simulink model "Open_Ciruit_Tests_of_Single_Phase_Transformer"  (R2025a)
settings: Solver=ode23tb  StartTime=0.0  StopTime=5  MaxStep=1e-4  RelTol=1e-3
libraries: spsRMSLib x2, spsCurrentMeasurementLib x1, spsLinearTransformerLib x1, spsPowerLib x1, spsVoltageMeasurementLib x1, spsACVoltageSourceLib x1, spspowerguiLib x1
settings Model: Creator=Jawad  LastModifiedBy=Jawad

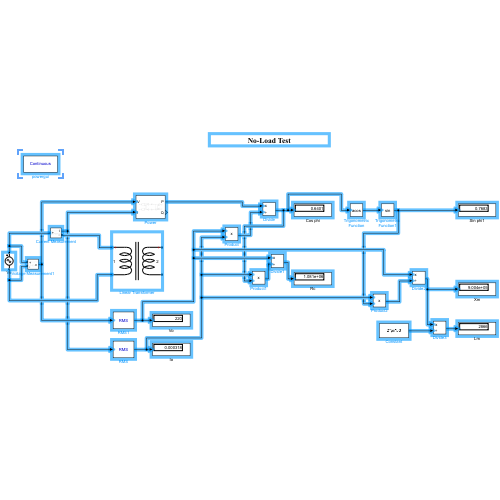
[thumbnail: Simulink's stored preview of the top-level diagram]
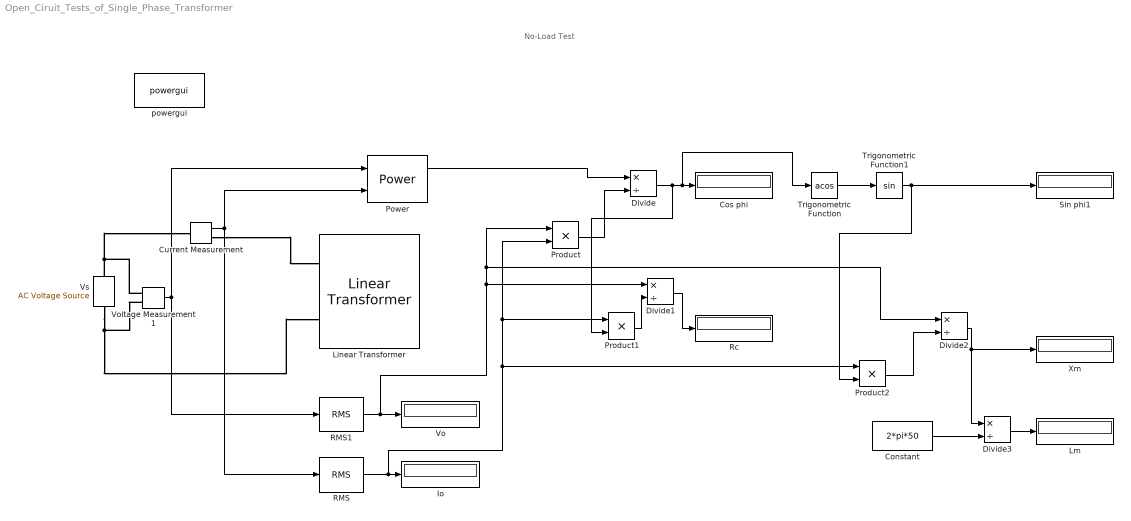
== system Open_Ciruit_Tests_of_Single_Phase_Transformer ==
  note: No-Load Test
  Constant : Constant  Value=2*pi*50
  Cos phi : Display
  Current Measurement : spsCurrentMeasurementLib/Current Measurement  PhasorSimulation=off  OutputType=Complex  PSBequivalent=0
  Divide{,1..3} (4 alike) : Product  Inputs=*/
  Io : Display
  Linear Transformer : spsLinearTransformerLib/Linear Transformer  UNITS=SI  NominalPower=[ 2000 50 ]  winding1=[220 4.3218 0.45856]  winding2=[110 0.7938 0.084225]  ThreeWindings=off  winding3=[3.15e+05 0.7938 0.084225]  RmLm=[1.0804e+06 2866]  Measurements=None  DataType=on
  Lm : Display
  Power : spsPowerLib/Power  Freq=50  Vinit=[1, 0]  Iinit=[1, 0]  Ts=0
  Product : Product
  Product1 : Product
  Product2 : Product
  RMS : spsRMSLib/RMS  TrueRMS=off  Freq=50  RMSInit=0  Ts=0
  RMS1 : spsRMSLib/RMS  TrueRMS=off  Freq=50  RMSInit=0  Ts=0
  Rc : Display
  Sin phi1 : Display
  Trigonometric Function : Trigonometry  Operator=acos
  Trigonometric Function1 : Trigonometry
  Vo : Display
  Voltage Measurement1 : spsVoltageMeasurementLib/Voltage Measurement  PhasorSimulation=off  OutputType=Complex  PSBequivalent=0
  Vs : spsACVoltageSourceLib/AC Voltage Source  Amplitude=220*sqrt(2)  Phase=0  Frequency=50  SampleTime=0  Measurements=None  BusType=swing  Pref=10e3  Qref=0  Qmin=-inf  Qmax=+inf
  Xm : Display
  powergui : spspowerguiLib/powergui  Priority=1  SimulationMode=Continuous  SampleTime=50e-6  frequency=60  Iterations=50  frequencyindice=50  Pbase=100e6  ErrMax=1e-4  UnitsV=kV  UnitsW=MW  buscounter=0  FunctionMessages=off  echomessages=off  EnableUseOfTLC=off  CurrentSourceSwitches=off  DisableSnubberDevices=off  DisableRonSwitches=off  DisableVfSwitches=off  DisplayEquations=off  AutomaticDiscreteSolvers=off  SolverType=Tustin/Backward Euler (TBE)  Interpol=off  ExternalGateDelay=off  methode=off  Ts=100  x0status=blocks  SPID=on  SwTol=0  HookPort=off  NonlinearTolerance=1e-4  nMaxIteration=100  ContinueOnMaxIteration=off  RestoreLinks=warning  ResistiveCurrentMeasurement=off  Frange=[0:2:500]  Ylog=off  Xlog=on  ShowGrid=off  save=off  variable=ZData  structure=0  ZoomFFT=off  StartTime=0.0  cycles=1  DisplayStyle=1  fundamental=60  FreqAxis=off  MaxFrequency=1000  frequencyindicesteady=1  RmsSteady=1  display=off
  wires:
  Current Measurement/1 -> RMS/1, Power/2
  Voltage Measurement1/1 -> RMS1/1, Power/1
  RMS/1 -> Product2/1, Product1/1, Product/2, Io/1
  Power/1 -> Divide/1
  Product/1 -> Divide/2
  RMS1/1 -> Divide1/1, Divide2/1, Product/1, Vo/1
  Divide/1 -> Product1/2, Trigonometric Function/1, Cos phi/1
  Product1/1 -> Divide1/2
  Divide1/1 -> Rc/1
  Trigonometric Function/1 -> Trigonometric Function1/1
  Trigonometric Function1/1 -> Product2/2, Sin phi1/1
  Product2/1 -> Divide2/2
  Divide2/1 -> Divide3/1, Xm/1
  Constant/1 -> Divide3/2
  Divide3/1 -> Lm/1
  connections:
  Vs/RConn1 -- Current Measurement/LConn1 -- Voltage Measurement1/LConn1
  Current Measurement/RConn1 -- Linear Transformer/LConn1
  Vs/LConn1 -- Voltage Measurement1/LConn2 -- Linear Transformer/LConn2
